simulink model "buck_06_2018_b"  (Simulink 9.2)
settings: Solver=ode15s  StartTime=0.0  StopTime=2000/F  MaxStep=1/(10*F)  RelTol=1e-3  EnableMultiTasking=on
values from neighbouring files (symbols this model uses):
  C = 9.3e-6    (= 9.3e-06)    [buck_01_script.m]    (also in buck_02_script.m; buck_04_script.m)
  C1 = 5.5e-6    (= 5.5e-06)    [buck_01_script.m]    (also in buck_02_script.m; buck_04_script.m)
  F = 500e3    (= 500000)    [buck_01_script.m]    (also in buck_02_script.m; buck_04_script.m)
  Kp = 10^(-50/20)    (= 0.00316227766017)    [buck_04_script.m]
  L = 1.9e-6    (= 1.9e-06)    [buck_01_script.m]    (also in buck_02_script.m; buck_04_script.m)
  L1 = 5e-6    (= 5e-06)    [buck_01_script.m]    (also in buck_02_script.m; buck_04_script.m)
  R = Vs^2 / Ps    (= 5.445)    [buck_01_script.m]    (also in buck_02_script.m = 0.5445; buck_04_script.m)
  Ti = 1e-6    (= 1e-06)    [buck_04_script.m]
  Ve = 5    [buck_01_script.m]    (also in buck_02_script.m; buck_04_script.m)
  Vs = 3.3    [buck_01_script.m]    (also in buck_02_script.m; buck_04_script.m)
libraries: powerlib x31, eePwmGenerator x1, simulink x1
settings Model: Creator=lefrancp  LastModifiedBy=lefrancp
settings DataIOCC: SaveFinalState=on  SignalLoggingSaveFormat=Dataset  SaveOutput=off
settings DebuggingCC: UnderspecifiedInitializationDetection=Simplified  MergeDetectMultiDrivingBlocksExec=error  SolverPrmCheckMsg=warning  FcnCallInpInsideContextMsg=error  StateNameClashWarn=none
settings GRTTargetCC: CombineOutputUpdateFcns=on  GRTInterface=off
settings ConfigComp: CovSFcnEnable=off
settings SimscapeCC: SimscapeNormalizeSystem=off

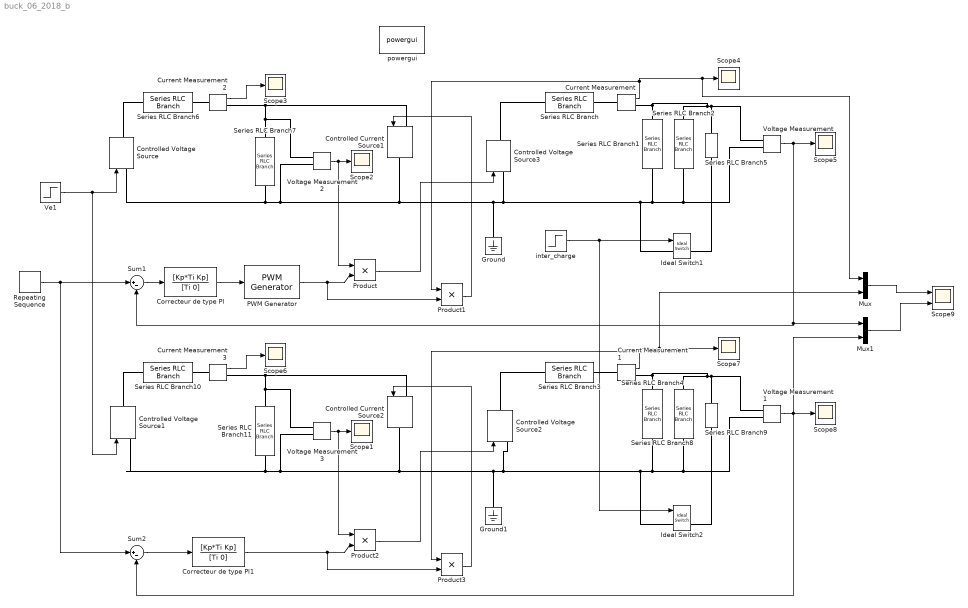
== system buck_06_2018_b ==
  Controlled Current Source1 : powerlib/Electrical Sources/Controlled Current Source  Initialize=on  Source_Type=AC  Amplitude=0  Phase=0  Frequency=0  Measurements=None
  Controlled Current Source2 : powerlib/Electrical Sources/Controlled Current Source  Initialize=on  Source_Type=AC  Amplitude=0  Phase=0  Frequency=0  Measurements=None
  Controlled Voltage Source{,1..3} (4 alike) : powerlib/Electrical Sources/Controlled Voltage Source  Initialize=on  Source_Type=AC  Amplitude=0  Phase=0  Frequency=0  Measurements=None
  Correcteur de type PI : TransferFcn  Numerator=[Kp*Ti Kp]  Denominator=[Ti 0]
  Correcteur de type PI1 : TransferFcn  Numerator=[Kp*Ti Kp]  Denominator=[Ti 0]
  Current Measurement{,1..3} (4 alike) : powerlib/Measurements/Current Measurement  PhasorSimulation=off  OutputType=Complex  PSBequivalent=0
  Ground : powerlib/Elements/Ground  LConnTagsString=a
  Ground1 : powerlib/Elements/Ground  LConnTagsString=a
  Ideal Switch1 : powerlib/Power Electronics/Ideal Switch  Ron=0.001  Lon=0  IC=0  Rs=1e5  Cs=inf  Measurements=on
  Ideal Switch2 : powerlib/Power Electronics/Ideal Switch  Ron=0.001  Lon=0  IC=0  Rs=1e5  Cs=inf  Measurements=on
  Mux : Mux  Inputs=2
  Mux1 : Mux  Inputs=2
  PWM Generator : eePwmGenerator/PWM Generator  CarrCount=Up  Tper=1/F  Ts=5e-9
  Product{,1..3} (4 alike) : Product
  Repeating Sequence : simulink/Sources/Repeating Sequence  rep_seq_t=[0 1e-3 10e-3]  rep_seq_y=[0 Vs Vs]
  Scope{1..8} (8 alike) : Scope
  Scope9 : Scope  NumInputPorts=2
  Series RLC Branch : powerlib/Elements/Series RLC Branch  LConnTagsString=__new0  RConnTagsString=__new0  BranchType=L  Resistance=1  Inductance=L  SetiL0=off  InitialCurrent=0  Capacitance=1e-6  Setx0=off  InitialVoltage=0  Measurements=None
  Series RLC Branch1 : powerlib/Elements/Series RLC Branch  LConnTagsString=__new0  RConnTagsString=__new0  BranchType=C  Resistance=1  Inductance=L  SetiL0=off  InitialCurrent=0  Capacitance=C  Setx0=off  InitialVoltage=0  Measurements=None
  Series RLC Branch10 : powerlib/Elements/Series RLC Branch  LConnTagsString=__new0  RConnTagsString=__new0  BranchType=L  Resistance=1  Inductance=L1  SetiL0=off  InitialCurrent=0  Capacitance=1e-6  Setx0=off  InitialVoltage=0  Measurements=None
  Series RLC Branch11 : powerlib/Elements/Series RLC Branch  LConnTagsString=__new0  RConnTagsString=__new0  BranchType=C  Resistance=1  Inductance=L  SetiL0=off  InitialCurrent=0  Capacitance=C1  Setx0=off  InitialVoltage=0  Measurements=None
  Series RLC Branch2 : powerlib/Elements/Series RLC Branch  LConnTagsString=__new0  RConnTagsString=__new0  BranchType=R  Resistance=R  Inductance=L  SetiL0=off  InitialCurrent=0  Capacitance=C  Setx0=off  InitialVoltage=0  Measurements=None
  Series RLC Branch3 : powerlib/Elements/Series RLC Branch  LConnTagsString=__new0  RConnTagsString=__new0  BranchType=L  Resistance=1  Inductance=L  SetiL0=off  InitialCurrent=0  Capacitance=1e-6  Setx0=off  InitialVoltage=0  Measurements=None
  Series RLC Branch4 : powerlib/Elements/Series RLC Branch  LConnTagsString=__new0  RConnTagsString=__new0  BranchType=C  Resistance=1  Inductance=L  SetiL0=off  InitialCurrent=0  Capacitance=C  Setx0=off  InitialVoltage=0  Measurements=None
  Series RLC Branch5 : powerlib/Elements/Series RLC Branch  LConnTagsString=__new0  RConnTagsString=__new0  BranchType=R  Resistance=R*5  Inductance=L  SetiL0=off  InitialCurrent=0  Capacitance=C  Setx0=off  InitialVoltage=0  Measurements=None
  Series RLC Branch6 : powerlib/Elements/Series RLC Branch  LConnTagsString=__new0  RConnTagsString=__new0  BranchType=L  Resistance=1  Inductance=L1  SetiL0=off  InitialCurrent=0  Capacitance=1e-6  Setx0=off  InitialVoltage=0  Measurements=None
  Series RLC Branch7 : powerlib/Elements/Series RLC Branch  LConnTagsString=__new0  RConnTagsString=__new0  BranchType=C  Resistance=1  Inductance=L  SetiL0=off  InitialCurrent=0  Capacitance=C1  Setx0=off  InitialVoltage=0  Measurements=None
  Series RLC Branch8 : powerlib/Elements/Series RLC Branch  LConnTagsString=__new0  RConnTagsString=__new0  BranchType=R  Resistance=R  Inductance=L  SetiL0=off  InitialCurrent=0  Capacitance=C  Setx0=off  InitialVoltage=0  Measurements=None
  Series RLC Branch9 : powerlib/Elements/Series RLC Branch  LConnTagsString=__new0  RConnTagsString=__new0  BranchType=R  Resistance=R*5  Inductance=L  SetiL0=off  InitialCurrent=0  Capacitance=C  Setx0=off  InitialVoltage=0  Measurements=None
  Sum1 : Sum  Inputs=|+-
  Sum2 : Sum  Inputs=|+-
  Ve1 : Step  Time=2e-3  Before=Ve  After=Ve+0.1  SampleTime=0
  Voltage Measurement{,1..3} (4 alike) : powerlib/Measurements/Voltage Measurement  PhasorSimulation=off  OutputType=Complex  PSBequivalent=0
  inter_charge : Step  Time=3e-3  SampleTime=0
  powergui : powerlib/powergui  Priority=1  SimulationMode=Continuous  SampleTime=50e-6  frequency=60  Iterations=50  frequencyindice=0  Pbase=100e6  ErrMax=1e-4  UnitsV=kV  UnitsW=MW  buscounter=0  FunctionMessages=off  echomessages=off  EnableUseOfTLC=off  CurrentSourceSwitches=on  DisableSnubberDevices=off  DisableRonSwitches=off  DisableVfSwitches=off  DisplayEquations=off  AutomaticDiscreteSolvers=off  SolverType=Tustin  Interpol=off  ExternalGateDelay=off  methode=off  Ts=0  x0status=blocks  SPID=off  SwTol=0  HookPort=off  NonlinearTolerance=0  nMaxIteration=15  ContinueOnMaxIteration=off  RestoreLinks=warning  ResistiveCurrentMeasurement=off  Frange=[0:2:500]  Ylog=off  Xlog=on  ShowGrid=off  save=off  variable=ZData  structure=0  ZoomFFT=off  StartTime=0.0  cycles=1  DisplayStyle=1  fundamental=60  FreqAxis=off  MaxFrequency=1000  frequencyindicesteady=1  RmsSteady=1  display=off
  wires:
  Voltage Measurement/1 -> Mux1/1, Sum1/2, Scope5/1
  Current Measurement/1 -> Product1/1, Mux/1, Scope4/1
  Voltage Measurement2/1 -> Product/1, Scope2/1
  Current Measurement2/1 -> Scope3/1
  Correcteur de type PI/1 -> PWM Generator/1
  Product/1 -> Controlled Voltage Source3/1
  Product1/1 -> Controlled Current Source1/1
  Sum1/1 -> Correcteur de type PI/1
  PWM Generator/1 -> Product1/2, Product/2
  Sum2/1 -> Correcteur de type PI1/1
  Product2/1 -> Controlled Voltage Source2/1
  Voltage Measurement3/1 -> Product2/1, Scope1/1
  Current Measurement1/1 -> Product3/1, Mux/2, Scope7/1
  Current Measurement3/1 -> Scope6/1
  Repeating Sequence/1 -> Sum2/1, Sum1/1
  Ve1/1 -> Controlled Voltage Source1/1, Controlled Voltage Source/1
  inter_charge/1 -> Ideal Switch2/1, Ideal Switch1/1
  Product3/1 -> Controlled Current Source2/1
  Correcteur de type PI1/1 -> Product3/2, Product2/2
  Voltage Measurement1/1 -> Mux1/2, Sum2/2, Scope8/1
  Mux/1 -> Scope9/1
  Mux1/1 -> Scope9/2
  connections:
  Ground/LConn1 -- Ideal Switch1/LConn1 -- Series RLC Branch1/RConn1 -- Voltage Measurement/LConn2 -- Series RLC Branch2/RConn1 -- Controlled Voltage Source3/LConn1 -- Controlled Current Source1/RConn1 -- Voltage Measurement2/LConn2 -- Series RLC Branch7/RConn1 -- Controlled Voltage Source/LConn1
  Controlled Voltage Source3/RConn1 -- Series RLC Branch/LConn1
  Series RLC Branch1/LConn1 -- Current Measurement/RConn1 -- Series RLC Branch5/LConn1 -- Voltage Measurement/LConn1 -- Series RLC Branch2/LConn1
  Series RLC Branch7/LConn1 -- Voltage Measurement2/LConn1 -- Controlled Current Source1/LConn1 -- Current Measurement2/RConn1
  Series RLC Branch/RConn1 -- Current Measurement/LConn1
  Series RLC Branch6/LConn1 -- Controlled Voltage Source/RConn1
  Current Measurement2/LConn1 -- Series RLC Branch6/RConn1
  Ideal Switch1/RConn1 -- Series RLC Branch5/RConn1
  Series RLC Branch4/RConn1 -- Ideal Switch2/LConn1 -- Ground1/LConn1 -- Controlled Current Source2/RConn1 -- Voltage Measurement3/LConn2 -- Series RLC Branch11/RConn1 -- Controlled Voltage Source1/LConn1 -- Controlled Voltage Source2/LConn1 -- Voltage Measurement1/LConn2 -- Series RLC Branch8/RConn1
  Current Measurement3/RConn1 -- Series RLC Branch11/LConn1 -- Voltage Measurement3/LConn1 -- Controlled Current Source2/LConn1
  Series RLC Branch8/LConn1 -- Series RLC Branch9/LConn1 -- Voltage Measurement1/LConn1 -- Series RLC Branch4/LConn1 -- Current Measurement1/RConn1
  Current Measurement3/LConn1 -- Series RLC Branch10/RConn1
  Series RLC Branch10/LConn1 -- Controlled Voltage Source1/RConn1
  Series RLC Branch3/RConn1 -- Current Measurement1/LConn1
  Controlled Voltage Source2/RConn1 -- Series RLC Branch3/LConn1
  Ideal Switch2/RConn1 -- Series RLC Branch9/RConn1
